simulink model "tractor_change_detection"  (R2024b)
settings: Solver=ode4  StartTime=0.0  StopTime=tStop  FixedStep=0.01  RelTol=1e-3
model workspace (MAT data in the model file):
  imuXRearAxleM = 0
  p0 = [10178.6; 1.6562; 1.1538; 19450.5265478; 356356.4449; 270000; 1.10369051]
  p1 = [10178.6; 1.6562; 1.1538; 19450.5265478; 356356.4449; 270000; 1.10369051]
  tEnd = 0
  tStart = 0
  tStop = 10
  x0_plant = [0; 0; 0; 0; 0; 0]
undefined symbols (not defined in the file or in its folder): useReplay
settings Model: Creator=Jhuessy  LastModifiedBy=Jhuessy

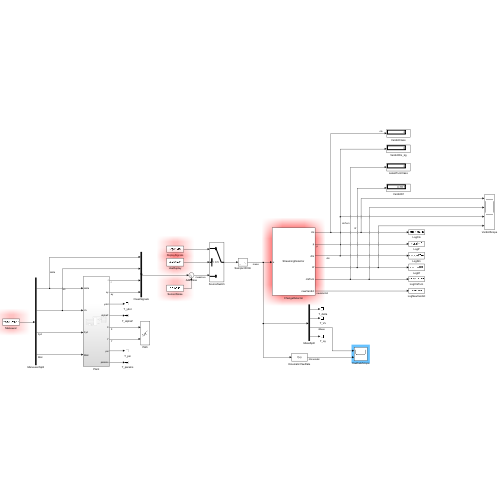
[thumbnail: Simulink's stored preview of the top-level diagram]
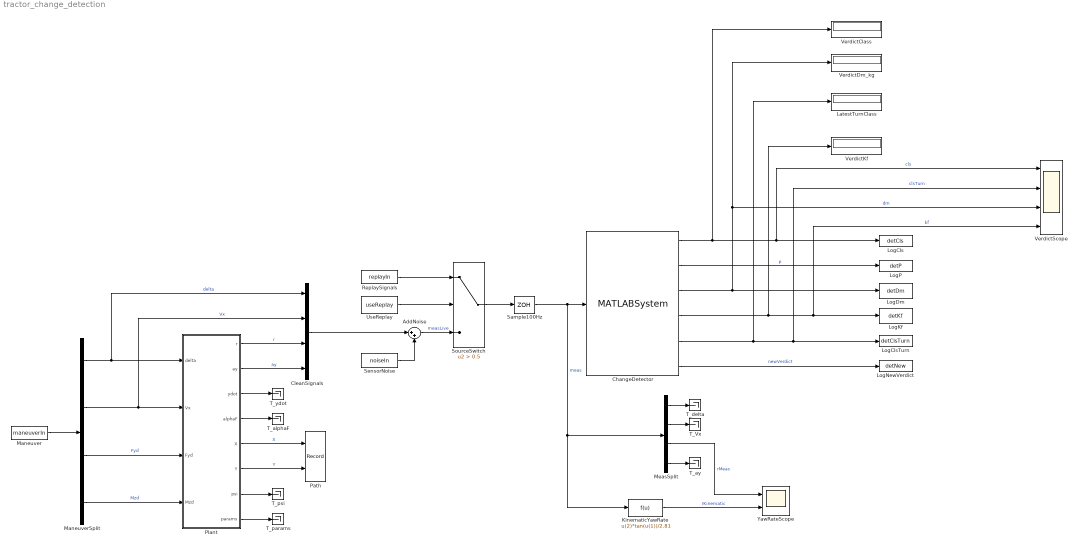
== system tractor_change_detection ==
  AddNoise : Sum  Inputs=|++
  ChangeDetector : MATLABSystem  System=change_detector.StreamingDetector  W=detW  fs=100  K=3  bufferS=150  SimulateUsing=Interpreted execution
      mask Type: change_detector.StreamingDetector
      mask Display:
      | disp('StreamingDetector');
      | port_label('input',1,'u');
      | port_label('output',1,'cls');
      | port_label('output',2,'p');
      | port_label('output',3,'dm');
      | port_label('output',4,'kf');
      | port_label('output',5,'clsTurn');
      | port_label('output',6,'newVerdict');
  CleanSignals : Mux
  KinematicYawRate : Fcn  Expr=u(2)*tan(u(1))/2.81
  LatestTurnClass : Display
  LogCls : ToWorkspace  VariableName=detCls  SampleTime=-1
      settings: Save2DSignal=2-D array (concatenate along first dimension)
  LogClsTurn : ToWorkspace  VariableName=detClsTurn  SampleTime=-1
      settings: Save2DSignal=2-D array (concatenate along first dimension)
  LogDm : ToWorkspace  VariableName=detDm  SampleTime=-1
      settings: Save2DSignal=2-D array (concatenate along first dimension)
  LogKf : ToWorkspace  VariableName=detKf  SampleTime=-1
      settings: Save2DSignal=2-D array (concatenate along first dimension)
  LogNewVerdict : ToWorkspace  VariableName=detNew  SampleTime=-1
      settings: Save2DSignal=2-D array (concatenate along first dimension)
  LogP : ToWorkspace  VariableName=detP  SampleTime=-1
      settings: Save2DSignal=2-D array (concatenate along first dimension)
  Maneuver : FromWorkspace  VariableName=maneuverIn  OutputAfterFinalValue=Holding final value
  ManeuverSplit : Demux
  MeasSplit : Demux
  Path : Record  FileSettingsInternal="{\"entries\":[{\"content\":{\"excelSettings\":{\"content\":{},\"type\":\"Streamout.ExcelSettings\"}},\"type\":\"Streamout.FileSettingStorage\",\"uuid\":\"\"}],\"packageUris\":[\"http:\\/\\/schema.mathworks.com\\/mf0\\/streamout_blocks\\/R2020a\"],\"version\":\"1.0\"}"  Layout=[1 1]  SignalsInternal="{\"entries\":[{\"content\":{\"signals\":[{\"content\":{\"blockPath\":[],\"dimensions\":[1],\"domain\":\"\",\"lineColor\":\"#a2142f\",\"plots\":[ 1 ],\"port\":1,\"sid\":[\"\"],\"signalID\":1,\"signalName\":\"X\"},\"type\":\"RecordBlkView.Signal\",\"uuid\":\"\"},{\"content\":{\"blockPath\":[],\"dimensions\":[1],\"domain\":\"\",\"lineColor\":\"#139fff\",\"plots\":[ 1 ],\"port\":2,\"sid\":[\"\"],\"signalID\":2,\"signalName\":\"Y\"},\"type\":\"RecordBlkView.Signal\",\"uuid\":\"\"}]},\"type\":\"RecordBlkView.InputSignals\",\"uuid\":\"\"}],\"packageUris\":[\"http:\\/\\/schema.mathworks.com\\/mf0\\/streamout_blocks\\/R2020a\"],\"version\":\"1.0\"}"  VisualizationBindings="{\"xyplotplugin\":{\"info\":[{\"series\":[{\"bindingParametersList\":[{\"parameter\":\"X-Axis\",\"signalID\":1,\"signalName\":\"X\"},{\"parameter\":\"Y-Axis\",\"signalID\":2,\"signalName\":\"Y\"}],\"seriesID\":0}],\"subplotID\":1}]}}"  CompatibilityTag=XY  st=-1
  Plant : Subsystem
  ReplaySignals : FromWorkspace  VariableName=replayIn  Interpolate=off  OutputAfterFinalValue=Holding final value
  Sample100Hz : ZeroOrderHold  SampleTime=0.01
  SensorNoise : FromWorkspace  VariableName=noiseIn  Interpolate=off  OutputAfterFinalValue=Holding final value
  SourceSwitch : Switch  Criteria=u2 > Threshold  Threshold=0.5
  T_Vx : Terminator
  T_alphaF : Terminator
  T_ay : Terminator
  T_delta : Terminator
  T_params : Terminator
  T_psi : Terminator
  T_ydot : Terminator
  UseReplay : Constant  Value=useReplay
  VerdictClass : Display
  VerdictDm_kg : Display
  VerdictKf : Display
  VerdictScope : Scope  NumInputPorts=4
  YawRateScope : Scope  NumInputPorts=2
  wires:
  ChangeDetector/2 -> LogP/1  "p"
  ManeuverSplit/4 -> Plant/4(Mzd)  "Mzd"
  AddNoise/1 -> SourceSwitch/3  "measLive"
  ManeuverSplit/3 -> Plant/3(Fyd)  "Fyd"
  ManeuverSplit/2 -> Plant/2(Vx), CleanSignals/2  "Vx"
  ManeuverSplit/1 -> Plant/1(delta), CleanSignals/1  "delta"
  Maneuver/1 -> ManeuverSplit/1
  Plant/3(ydot) -> T_ydot/1
  Plant/2(ay) -> CleanSignals/4  "ay"
  Plant/1(r) -> CleanSignals/3  "r"
  Plant/4(alphaF) -> T_alphaF/1
  Plant/5(X) -> Path/1  "X"
  KinematicYawRate/1 -> YawRateScope/2  "rKinematic"
  Plant/6(Y) -> Path/2  "Y"
  Plant/7(psi) -> T_psi/1
  MeasSplit/4 -> T_ay/1
  Plant/8(params) -> T_params/1
  SensorNoise/1 -> AddNoise/2
  CleanSignals/1 -> AddNoise/1
  ChangeDetector/5 -> VerdictScope/2, LogClsTurn/1, LatestTurnClass/1  "clsTurn"
  ReplaySignals/1 -> SourceSwitch/1
  UseReplay/1 -> SourceSwitch/2
  SourceSwitch/1 -> Sample100Hz/1
  Sample100Hz/1 -> KinematicYawRate/1, MeasSplit/1, ChangeDetector/1  "meas"
  ChangeDetector/1 -> VerdictClass/1, VerdictScope/1, LogCls/1  "cls"
  ChangeDetector/3 -> LogDm/1, VerdictDm_kg/1, VerdictScope/3  "dm"
  ChangeDetector/4 -> LogKf/1, VerdictScope/4, VerdictKf/1  "kf"
  ChangeDetector/6 -> LogNewVerdict/1  "newVerdict"
  MeasSplit/1 -> T_delta/1
  MeasSplit/2 -> T_Vx/1
  MeasSplit/3 -> YawRateScope/1  "rMeas"

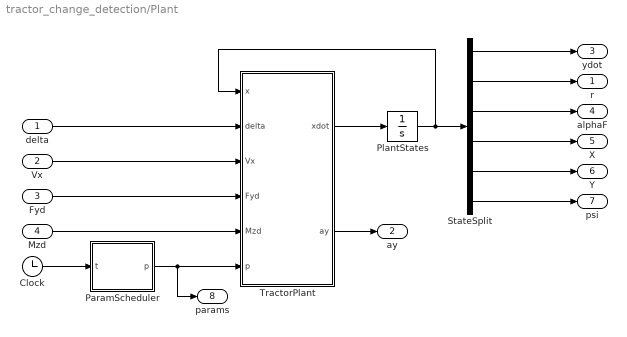
== system tractor_change_detection/Plant ==
  delta : Inport
  Vx : Inport  Port=2
  Fyd : Inport  Port=3
  Mzd : Inport  Port=4
  Clock : Clock
  ParamScheduler : MATLAB Function  TreatAsAtomicUnit=on
  PlantStates : Integrator  InitialCondition=x0_plant
  StateSplit : Demux  Outputs=6
  TractorPlant : MATLAB Function  TreatAsAtomicUnit=on
  r : Outport
  ay : Outport  Port=2
  ydot : Outport  Port=3
  alphaF : Outport  Port=4
  X : Outport  Port=5
  Y : Outport  Port=6
  psi : Outport  Port=7
  params : Outport  Port=8
  wires:
  Clock/1 -> ParamScheduler/1(t)
  ParamScheduler/1(p) -> TractorPlant/6(p), params/1
  PlantStates/1 -> StateSplit/1, TractorPlant/1(x)
  delta/1 -> TractorPlant/2(delta)
  Vx/1 -> TractorPlant/3(Vx)
  Fyd/1 -> TractorPlant/4(Fyd)
  Mzd/1 -> TractorPlant/5(Mzd)
  TractorPlant/1(xdot) -> PlantStates/1
  TractorPlant/2(ay) -> ay/1
  StateSplit/1 -> ydot/1
  StateSplit/2 -> r/1
  StateSplit/3 -> alphaF/1
  StateSplit/4 -> X/1
  StateSplit/5 -> Y/1
  StateSplit/6 -> psi/1

== matlab function tractor_change_detection/Plant/TractorPlant ==
  data: x input; xdot output size=6; delta input; Vx input; Fyd input; Mzd input; p input; ay output; imuXRearAxleM parameter
function [xdot, ay] = fcn(x, delta, Vx, Fyd, Mzd, p, imuXRearAxleM)

% x = [ydot; r; alphaF; X; Y; psi], p = [m lf lr Izz Caf Car sigmaF]
m = p(1); lf = p(2); lr = p(3); Izz = p(4); Caf = p(5); Car = p(6); sig = p(7);

v = x(1); r = x(2); af = x(3); psi = x(6);

Fyf = Caf*af;
Fyr = -Car*(v - lr*r)/Vx;

vdot = (Fyf + Fyr + Fyd)/m - Vx*r;
rdot = (lf*Fyf - lr*Fyr + Mzd)/Izz;
afdot = (Vx*delta - v - lf*r - Vx*af)/sig;
xdot = [vdot; rdot; afdot; Vx*cos(psi) - v*sin(psi); Vx*sin(psi) + v*cos(psi); r];

% IMU is fixed to the chassis at imuXRearAxleM ahead of the rear axle, i.e. (imuXRearAxleM - lr) ahead of the CG
ay = vdot + Vx*r + (imuXRearAxleM - lr)*rdot;

== matlab function tractor_change_detection/Plant/ParamScheduler ==
  data: t input; p output size=7; p0 parameter; p1 parameter; tStart parameter; tEnd parameter
function p = fcn(t, p0, p1, tStart, tEnd)
% Blend nominal parameters p0 into p1 between tStart and tEnd (step if tEnd ~ tStart).
% p = [m lf lr Izz Caf Car sigmaF]
s = min(max((t - tStart)/max(tEnd - tStart, 1e-6), 0), 1);
p = p0 + s*(p1 - p0);
